simulink model "simula"  (R2013b)
settings: Solver=ode45  StartTime=0.0  StopTime=5  RelTol=1e-3
values from neighbouring files (symbols this model uses):
  beta = 15    [identifica3.m]
  dC = conv([0.065 1],[ 0.015 1])    [identifica3.m]
  gama = 0.7    [identifica3.m]
  KD = 2    [identifica3.m]
  KP = 18    [identifica3.m]
  nC = [0.12^2 0.21 1]    [identifica3.m]
  nG = sum(nG)    [identifica3.m]
  num = num(end)    [identifica3.m]
  T = 0.01    [identifica3.m]
undefined symbols (not defined in the file or in its folder): den, dG
settings Model: Creator=Guilherme  LastModifiedBy=Guilherme

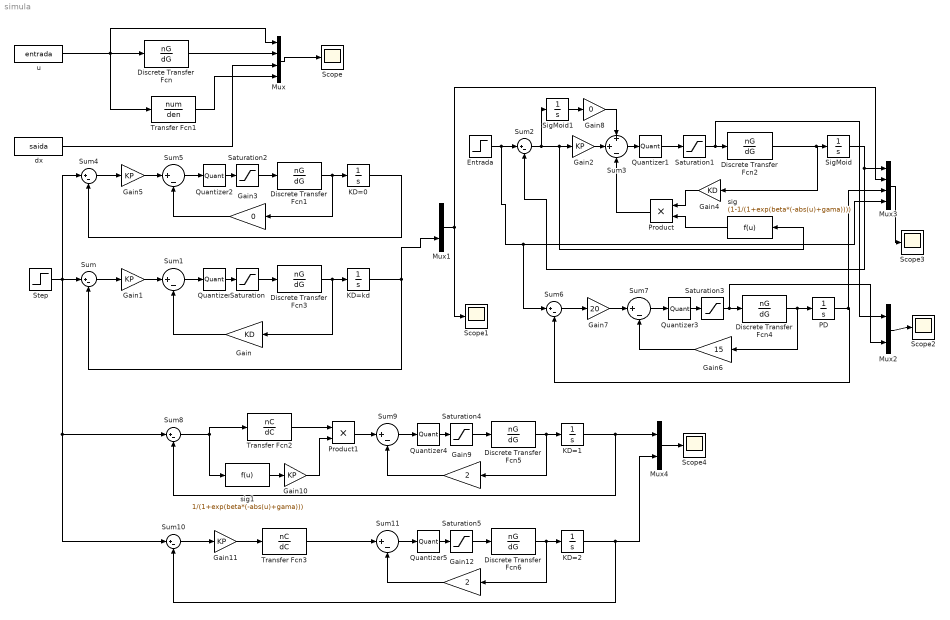
== system simula ==
  Discrete Transfer Fcn{,1..6} (7 alike) : DiscreteTransferFcn  Numerator=nG  Denominator=dG  SampleTime=T
  Entrada : Step  Time=0.5  SampleTime=0
  Gain : Gain  Gain=KD
  Gain{1..2,5,10..11} (5 alike) : Gain  Gain=KP
  Gain12 : Gain  Gain=2
  Gain3 : Gain  Gain=0
  Gain4 : Gain  Gain=KD
  Gain6 : Gain  Gain=15
  Gain7 : Gain  Gain=20
  Gain8 : Gain  Gain=0
  Gain9 : Gain  Gain=2
  KD=0 : Integrator
  KD=1 : Integrator
  KD=2 : Integrator
  KD=kd : Integrator
  Mux : Mux
  Mux1 : Mux  Inputs=2
  Mux2 : Mux  Inputs=2
  Mux3 : Mux
  Mux4 : Mux  Inputs=2
  PD : Integrator
  Product : Product
  Product1 : Product
  Quantizer{,1..5} (6 alike) : Quantizer  QuantizationInterval=1  SampleTime=T
  Saturation{,1..5} (6 alike) : Saturate  UpperLimit=50  LowerLimit=-50  SampleTime=T
  Scope{,1..4} (5 alike) : Scope
      Scope settings: MaxDataPoints=20000
      Scope1 settings: TimeRange=4  YMin=0  YMax=1.4
      Scope2 settings: ShowLegends=on  TimeRange=5  YMin=-50  YMax=30  SaveName=ScopeData2
      Scope3 settings: ShowLegends=on  TimeRange=5  YMin=0  YMax=1.4  SaveName=ScopeData3
      Scope4 settings: ShowLegends=on  TimeRange=5  YMin=-50  YMax=30  SaveName=ScopeData4
  SigMoid : Integrator
  SigMoid1 : Integrator
  Step : Step  Time=0.5  SampleTime=0
  Sum{,1..2,4..11} (11 alike) : Sum  Inputs=|+-
  Sum3 : Sum  Inputs=+|+|-
  Transfer Fcn1 : TransferFcn  Numerator=num  Denominator=den
  Transfer Fcn2 : TransferFcn  Numerator=nC  Denominator=dC
  Transfer Fcn3 : TransferFcn  Numerator=nC  Denominator=dC
  dx : FromWorkspace  VariableName=saida  SampleTime=T
  sig : Fcn  Expr=(1-1/(1+exp(beta*(-abs(u)+gama))))  SampleTime=T
  sig1 : Fcn  Expr=1/(1+exp(beta*(-abs(u)+gama)))  SampleTime=T
  u : FromWorkspace  VariableName=entrada  SampleTime=T
  wires:
  u/1 -> Transfer Fcn1/1, Mux/1, Discrete Transfer Fcn/1
  Mux/1 -> Scope/1
  Discrete Transfer Fcn/1 -> Mux/2
  dx/1 -> Mux/3
  Discrete Transfer Fcn3/1 -> Gain/1, KD=kd/1
  Sum/1 -> Gain1/1
  KD=kd/1 -> Sum/2, Mux1/2
  Sum1/1 -> Quantizer/1
  Mux1/1 -> Scope1/1, Mux3/2
  Quantizer/1 -> Saturation/1
  Saturation/1 -> Discrete Transfer Fcn3/1
  Transfer Fcn1/1 -> Mux/4
  Quantizer1/1 -> Saturation1/1
  Entrada/1 -> Mux3/4, Sum6/1, Sum2/1
  Gain2/1 -> Sum3/2
  Sum3/1 -> Quantizer1/1
  Saturation1/1 -> Mux2/1, Discrete Transfer Fcn2/1
  SigMoid/1 -> Mux3/1, Sum2/2
  Gain/1 -> Sum1/2
  Mux3/1 -> Scope3/1
  sig/1 -> Product/2
  Gain4/1 -> Product/1
  Gain1/1 -> Sum1/1
  Discrete Transfer Fcn1/1 -> Gain3/1, KD=0/1
  Sum4/1 -> Gain5/1
  KD=0/1 -> Sum4/2
  Sum5/1 -> Quantizer2/1
  Quantizer2/1 -> Saturation2/1
  Saturation2/1 -> Discrete Transfer Fcn1/1
  Gain3/1 -> Sum5/2
  Gain5/1 -> Sum5/1
  Discrete Transfer Fcn4/1 -> Gain6/1, PD/1
  Sum6/1 -> Gain7/1
  PD/1 -> Mux3/3, Sum6/2
  Sum7/1 -> Quantizer3/1
  Quantizer3/1 -> Saturation3/1
  Saturation3/1 -> Mux2/2, Discrete Transfer Fcn4/1
  Gain6/1 -> Sum7/2
  Gain7/1 -> Sum7/1
  Discrete Transfer Fcn2/1 -> Gain4/1, SigMoid/1
  Product/1 -> Sum3/3
  Gain8/1 -> Sum3/1
  SigMoid1/1 -> Gain8/1
  Sum2/1 -> SigMoid1/1, sig/1, Gain2/1
  Mux2/1 -> Scope2/1
  Step/1 -> Sum10/1, Sum8/1, Sum4/1, Sum/1
  Discrete Transfer Fcn5/1 -> Gain9/1, KD=1/1
  Sum8/1 -> sig1/1, Transfer Fcn2/1
  KD=1/1 -> Mux4/1, Sum8/2
  Sum9/1 -> Quantizer4/1
  Quantizer4/1 -> Saturation4/1
  Saturation4/1 -> Discrete Transfer Fcn5/1
  Gain9/1 -> Sum9/2
  Transfer Fcn2/1 -> Product1/1
  Product1/1 -> Sum9/1
  sig1/1 -> Gain10/1
  Gain10/1 -> Product1/2
  Discrete Transfer Fcn6/1 -> Gain12/1, KD=2/1
  Sum10/1 -> Gain11/1
  KD=2/1 -> Mux4/2, Sum10/2
  Sum11/1 -> Quantizer5/1
  Quantizer5/1 -> Saturation5/1
  Saturation5/1 -> Discrete Transfer Fcn6/1
  Gain12/1 -> Sum11/2
  Gain11/1 -> Transfer Fcn3/1
  Transfer Fcn3/1 -> Sum11/1
  Mux4/1 -> Scope4/1
